simulink model "DC_LINK_VOLTAGE"  (R2023a)
settings: Solver=VariableStepAuto  StartTime=0.0  StopTime=2.0  RelTol=1e-3
libraries: spspowerguiLib x1
settings Model: Creator=Anikait  LastModifiedBy=Anikait

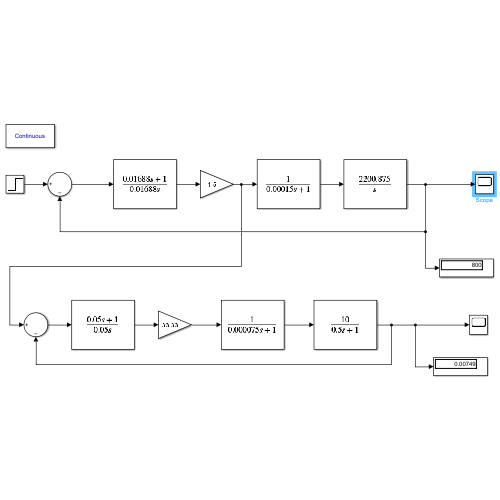
[thumbnail: Simulink's stored preview of the top-level diagram]
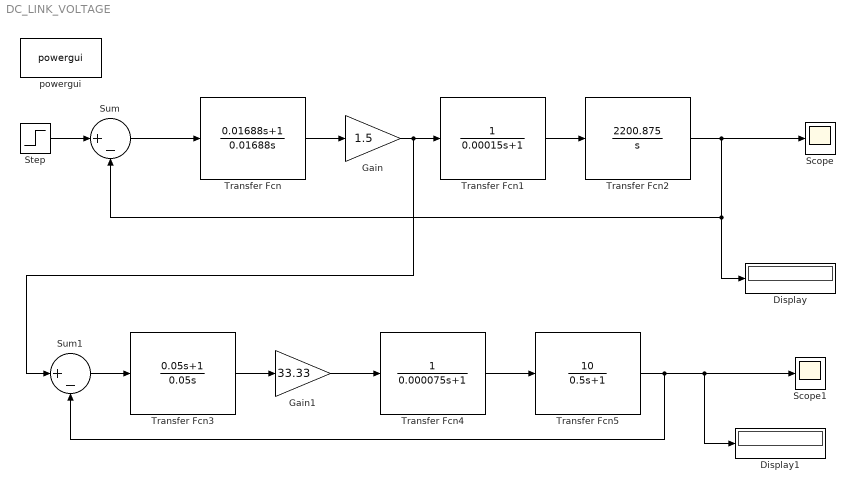
== system DC_LINK_VOLTAGE ==
  Display : Display
  Display1 : Display
  Gain : Gain  Gain=1.5
  Gain1 : Gain  Gain=33.33
  Scope : Scope
  Scope1 : Scope
  Step : Step  Before=400  After=800  SampleTime=0
  Sum : Sum  Inputs=|+-
  Sum1 : Sum  Inputs=|+-
  Transfer Fcn : TransferFcn  Numerator=[0.01688 1]  Denominator=[0.01688 0]
  Transfer Fcn1 : TransferFcn  Denominator=[0.00015 1]
  Transfer Fcn2 : TransferFcn  Numerator=[2200.875]  Denominator=[1 0]
  Transfer Fcn3 : TransferFcn  Numerator=[0.05 1]  Denominator=[0.05 0]
  Transfer Fcn4 : TransferFcn  Denominator=[0.000075 1]
  Transfer Fcn5 : TransferFcn  Numerator=[10]  Denominator=[0.5 1]
  powergui : spspowerguiLib/powergui  Priority=1  SimulationMode=Continuous  SampleTime=50e-6  frequency=60  Iterations=50  frequencyindice=60  Pbase=100e6  ErrMax=1e-4  UnitsV=kV  UnitsW=MW  buscounter=0  FunctionMessages=off  echomessages=off  EnableUseOfTLC=off  CurrentSourceSwitches=off  DisableSnubberDevices=off  DisableRonSwitches=off  DisableVfSwitches=off  DisplayEquations=off  AutomaticDiscreteSolvers=off  SolverType=Tustin/Backward Euler (TBE)  Interpol=off  ExternalGateDelay=off  methode=off  Ts=100  x0status=blocks  SPID=on  SwTol=0  HookPort=off  NonlinearTolerance=1e-4  nMaxIteration=100  ContinueOnMaxIteration=off  RestoreLinks=warning  ResistiveCurrentMeasurement=off  Frange=[0:2:500]  Ylog=off  Xlog=on  ShowGrid=off  save=off  variable=ZData  structure=0  ZoomFFT=off  StartTime=0.0  cycles=1  DisplayStyle=1  fundamental=60  FreqAxis=off  MaxFrequency=1000  frequencyindicesteady=1  RmsSteady=1  display=off
  wires:
  Transfer Fcn/1 -> Gain/1
  Transfer Fcn1/1 -> Transfer Fcn2/1
  Transfer Fcn2/1 -> Scope/1, Display/1, Sum/2
  Sum/1 -> Transfer Fcn/1
  Transfer Fcn3/1 -> Gain1/1
  Gain1/1 -> Transfer Fcn4/1
  Transfer Fcn4/1 -> Transfer Fcn5/1
  Transfer Fcn5/1 -> Display1/1, Scope1/1, Sum1/2
  Sum1/1 -> Transfer Fcn3/1
  Gain/1 -> Sum1/1, Transfer Fcn1/1
  Step/1 -> Sum/1
